simulink model "Asynchronous_Machine"  (R2023b)
settings: Solver=ode23s  StartTime=0.0  StopTime=10.0  MaxStep=1e-3  RelTol=1e-3
libraries: spsControlledVoltageSourceLib x3, spsAsynchronousMachineSIUnitsLib x1, simulink x1, spsVoltageMeasurementLib x1, sps_lib x1
settings Model: Creator=yello  LastModifiedBy=yello

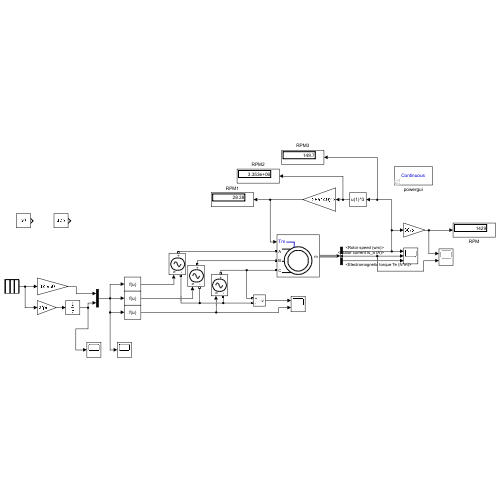
[thumbnail: Simulink's stored preview of the top-level diagram]
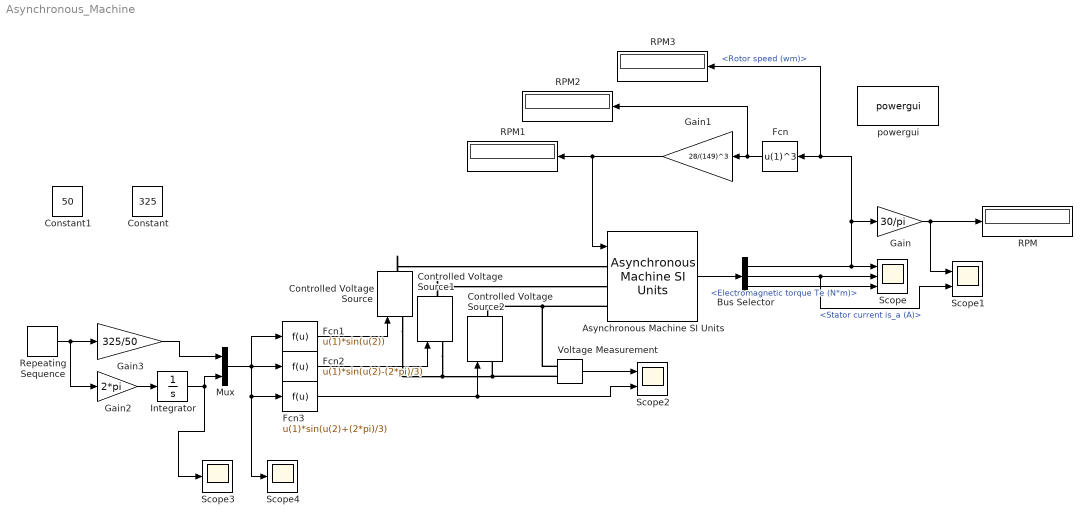
== system Asynchronous_Machine ==
  Asynchronous Machine SI Units : spsAsynchronousMachineSIUnitsLib/Asynchronous Machine SI Units  RotorType=Squirrel-cage  PresetModel="15:  5.4 HP (4KW)   400 V  50Hz 1430 RPM"  MechanicalLoad=Torque Tm  ShowDetailedParameters=on  ReferenceFrame=Rotor  Units=SI  MeasurementBus=off  NominalParameters=[4000 400 50]  VoltageRatio=1  Stator=[1.405 0.005839]  Rotor=[1.395 0.005839]  Cage1=[0.4155 0.002066]  Cage2=[0.4168 0.0003495]  Lm=0.1722  Mechanical=[0.0131 0.002985 2]  PolePairs=2  InitialConditions=[1 0 0 0 0 0 0 0]  SimulateSaturation=off  Saturation=[14.03593122, 27.81365428, 53.79336849, 72.68890987, 97.98006896, 148.6815601, 215.7428561, 302.9841135, 428.7778367 ; 230, 322, 414, 460, 506, 552, 598, 644, 690]  LoadFlowParameters=1492000  TsPowergui=0  TsBlock=-1  IterativeModel=Trapezoidal non iterative  IterativeDiscreteModel=Trapezoidal non iterative  Pmec=1.492e+006
  Bus Selector : BusSelector  OutputSignals=Mechanical.Rotor speed (wm),Stator measurements.Stator current is_a (A),Mechanical.Electromagnetic torque Te (N*m)
  Constant : Constant  Value=325
  Constant1 : Constant  Value=50
  Controlled Voltage Source : spsControlledVoltageSourceLib/Controlled Voltage Source  Initialize=on  Source_Type=AC  Amplitude=0  Phase=0  Frequency=0  Measurements=None
  Controlled Voltage Source1 : spsControlledVoltageSourceLib/Controlled Voltage Source  Initialize=on  Source_Type=AC  Amplitude=0  Phase=0  Frequency=0  Measurements=None
  Controlled Voltage Source2 : spsControlledVoltageSourceLib/Controlled Voltage Source  Initialize=on  Source_Type=AC  Amplitude=0  Phase=0  Frequency=0  Measurements=None
  Fcn : Fcn  Expr=u(1)^3
  Fcn1 : Fcn  Expr=u(1)*sin(u(2))
  Fcn2 : Fcn  Expr=u(1)*sin(u(2)-(2*pi)/3)
  Fcn3 : Fcn  Expr=u(1)*sin(u(2)+(2*pi)/3)
  Gain : Gain  Gain=30/pi
  Gain1 : Gain  Gain=28/(149)^3
  Gain2 : Gain  Gain=2*pi
  Gain3 : Gain  Gain=325/50
  Integrator : Integrator
  Mux : Mux  Inputs=2
  RPM{,1..3} (4 alike) : Display
  Repeating Sequence : simulink/Sources/Repeating Sequence  rep_seq_t=[0 .1 10]  rep_seq_y=[0 50 50]
  Scope : Scope  NumInputPorts=3
  Scope1 : Scope  NumInputPorts=2
  Scope2 : Scope  NumInputPorts=2
  Scope3 : Scope
  Scope4 : Scope
  Voltage Measurement : spsVoltageMeasurementLib/Voltage Measurement  PhasorSimulation=off  OutputType=Complex  PSBequivalent=0
  powergui : sps_lib/powergui  Priority=1  SimulationMode=Continuous  SampleTime=50e-6  frequency=60  Iterations=50  frequencyindice=50  Pbase=100e6  ErrMax=1e-4  UnitsV=kV  UnitsW=MW  buscounter=0  FunctionMessages=off  echomessages=off  EnableUseOfTLC=off  CurrentSourceSwitches=off  DisableSnubberDevices=off  DisableRonSwitches=off  DisableVfSwitches=off  DisplayEquations=off  AutomaticDiscreteSolvers=off  SolverType=Tustin/Backward Euler (TBE)  Interpol=off  ExternalGateDelay=off  methode=off  Ts=100  x0status=blocks  SPID=on  SwTol=0  HookPort=off  NonlinearTolerance=1e-4  nMaxIteration=100  ContinueOnMaxIteration=off  RestoreLinks=warning  ResistiveCurrentMeasurement=off  Frange=[0:2:500]  Ylog=off  Xlog=on  ShowGrid=off  save=off  variable=ZData  structure=0  ZoomFFT=off  StartTime=0.0  cycles=1  DisplayStyle=1  fundamental=60  FreqAxis=off  MaxFrequency=1000  frequencyindicesteady=1  RmsSteady=1  display=off
  wires:
  Asynchronous Machine SI Units/1 -> Bus Selector/1
  Bus Selector/2 -> Scope/2, Scope1/2  "<Stator current is_a (A)>"
  Bus Selector/1 -> RPM3/1, Fcn/1, Gain/1, Scope/1  "<Rotor speed (wm)>"
  Gain/1 -> Scope1/1, RPM/1
  Gain1/1 -> RPM1/1, Asynchronous Machine SI Units/1
  Fcn/1 -> RPM2/1, Gain1/1
  Voltage Measurement/1 -> Scope2/1
  Bus Selector/3 -> Scope/3  "<Electromagnetic torque Te (N*m)>"
  Fcn1/1 -> Controlled Voltage Source/1
  Fcn2/1 -> Controlled Voltage Source1/1
  Fcn3/1 -> Scope2/2, Controlled Voltage Source2/1
  Mux/1 -> Scope4/1, Fcn3/1, Fcn1/1, Fcn2/1
  Gain2/1 -> Integrator/1
  Integrator/1 -> Scope3/1, Mux/2
  Repeating Sequence/1 -> Gain2/1, Gain3/1
  Gain3/1 -> Mux/1
  connections:
  Controlled Voltage Source/RConn1 -- Asynchronous Machine SI Units/LConn1
  Controlled Voltage Source1/RConn1 -- Asynchronous Machine SI Units/LConn2
  Asynchronous Machine SI Units/LConn3 -- Voltage Measurement/LConn1 -- Controlled Voltage Source2/RConn1
  Controlled Voltage Source/LConn1 -- Controlled Voltage Source1/LConn1 -- Voltage Measurement/LConn2 -- Controlled Voltage Source2/LConn1
